simulink model "IC_surfaceTilt"  (R2015a)
settings: Solver=ode5  SolverMode=SingleTasking  StartTime=0  StopTime=sim_time-1/sr  FixedStep=1/sr  MaxStep=0.01  RelTol=1e-3  AbsTol=1e-3
values from neighbouring files (symbols this model uses):
  par = p.Results.par_fix    [balance_sim.m]
CloseFcn:
  | ;slview('closediagram',bdroot);;slview('closediagram',bdroot);
settings Model: ExtModeAutoUpdateStatusClock=off  Creator=bobbo  LastModifiedBy=lorenz
settings DataIOCC: LimitDataPoints=off  SignalLoggingSaveFormat=ModelDataLogs  SaveOutput=off  SaveTime=off
settings OptimizationCC: BlockReduction=off  BooleanDataType=off  ExpressionDepthLimit=2147483647  InitFltsAndDblsToZero=on
settings DebuggingCC: SaveWithParameterizedLinksMsg=none  UnderspecifiedInitializationDetection=Classic  MergeDetectMultiDrivingBlocksExec=none  SignalResolutionControl=TryResolveAllWithWarning  MultiTaskDSMMsg=warning  MultiTaskCondExecSysMsg=none  FcnCallInpInsideContextMsg=UseLocalSettings  StateNameClashWarn=warning  StrictBusMsg=None
settings HardwareCC: TargetUnknown=on
settings RTWCC: TemplateMakefile=grt_unix.tmf
settings GRTTargetCC: TargetFcnLib=ansi_tfl_tmw.mat  ModelReferenceCompliant=off  CombineOutputUpdateFcns=off  MatFileLogging=off  GRTInterface=on

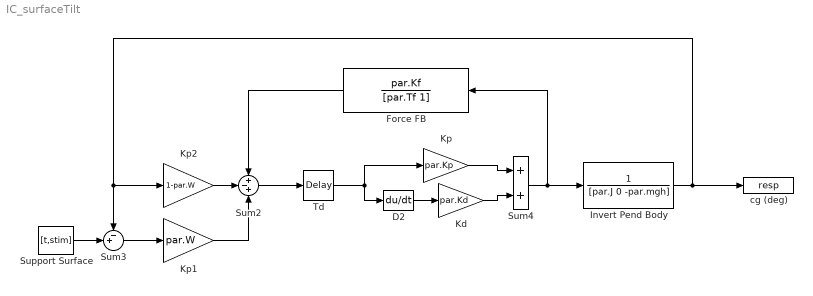
== system IC_surfaceTilt ==
  D2 : Derivative
  Force FB : TransferFcn  Numerator=par.Kf  Denominator=[par.Tf 1]
  Invert Pend Body : TransferFcn  Denominator=[par.J 0 -par.mgh]
  Kd : Gain  Gain=par.Kd  SaturateOnIntegerOverflow=on  OutDataTypeStr=Inherit: Same as input  ParamDataTypeStr=Inherit: Same as input
  Kp : Gain  Gain=par.Kp  SaturateOnIntegerOverflow=on  OutDataTypeStr=Inherit: Same as input  ParamDataTypeStr=Inherit: Same as input
  Kp1 : Gain  Gain=par.W  SaturateOnIntegerOverflow=on  OutDataTypeStr=Inherit: Same as input  ParamDataTypeStr=Inherit: Same as input
  Kp2 : Gain  Gain=1-par.W  SaturateOnIntegerOverflow=on  OutDataTypeStr=Inherit: Same as input  ParamDataTypeStr=Inherit: Same as input
  Sum2 : Sum  Inputs=+-+  SaturateOnIntegerOverflow=on  InputSameDT=on  OutDataTypeStr=Inherit: Same as first input
  Sum3 : Sum  Inputs=-+|  SaturateOnIntegerOverflow=on  InputSameDT=on  OutDataTypeStr=Inherit: Same as first input
  Sum4 : Sum  SaturateOnIntegerOverflow=on  InputSameDT=on  OutDataTypeStr=Inherit: Same as first input
  Support Surface : FromWorkspace  VariableName=[t,stim]  SampleTime=0
  Td : TransportDelay  DelayTime=par.dt
  cg (deg) : ToWorkspace  VariableName=resp  SampleTime=-1
  wires:
  Sum2/1 -> Td/1
  Support Surface/1 -> Sum3/2
  Force FB/1 -> Sum2/1
  Kp1/1 -> Sum2/3
  Sum3/1 -> Kp1/1
  Invert Pend Body/1 -> cg (deg)/1, Kp2/1, Sum3/1
  Sum4/1 -> Invert Pend Body/1, Force FB/1
  Kd/1 -> Sum4/2
  D2/1 -> Kd/1
  Kp/1 -> Sum4/1
  Td/1 -> Kp/1, D2/1
  Kp2/1 -> Sum2/2
